simulink model "RightCameraAgent"  (Simulink 6.2)
settings: Solver=ode45  StartTime=0.0  StopTime=10.0  RelTol=1e-3
settings Model: LastModifiedBy=suarezjl
settings DataIOCC: SignalLoggingName=sigsOut
settings HardwareCC: TargetUnknown=on

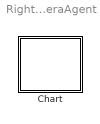
== system RightCameraAgent ==
  Chart : Stateflow chart

== stateflow chart Chart ==
  state Initial
    \\Sally\HeadTrackingDemo\HeadModule\RightCameraAgent\FrameGrabber.Initialize()
    \\Sally\HeadTrackingDemo\HeadModule\RightCameraAgent\FrameGrabber.ObtainImage()
    \\Sally\HeadTrackingDemo\HeadModule\RightCameraAgent\FrameGrabber.ObtainImage()
    \\Sally\HeadTrackingDemo\HeadModule\RightCameraAgent\ColorSegmenter.Initialize()
  state Segmentation
    \\Sally\HeadTrackingDemo\HeadModule\RightCameraAgent\FrameGrabber.ObtainImage()
    \\Sally\HeadTrackingDemo\HeadModule\RightCameraAgent\ColorSegmenter.DoSegment()
  (default) -> Initial : Start
  Initial -> Segmentation : Always
  Segmentation -> Segmentation : Always
